simulink model "TestModel2"  (R2012b)
settings: Solver=ode45  SolverMode=SingleTasking  StartTime=0.0  StopTime=10.0  RelTol=1e-3
libraries: simulink x3
settings Model: Creator=odj  LastModifiedBy=TSR2
settings DataIOCC: SignalLoggingSaveFormat=ModelDataLogs
settings OptimizationCC: BlockReduction=off  BooleanDataType=off
settings DebuggingCC: SaveWithParameterizedLinksMsg=none  SignalResolutionControl=TryResolveAllWithWarning  SolverPrmCheckMsg=none  MultiTaskDSMMsg=warning  MultiTaskCondExecSysMsg=none  StrictBusMsg=None
settings HardwareCC: TargetIntDivRoundTo=Zero  TargetEndianess=LittleEndian  TargetHWDeviceType=MATLAB Host  ProdEqTarget=off
settings RTWCC: SystemTargetFile=rtwsfcnfmi.tlc  TemplateMakefile=rtwsfcnfmi_tmf  Description=S-Function Target with Functional Mockup Interface (FMI)  ProcessScript=rtwsfcnfmi_make_rtw_hook  IncludeERTFirstTime=on
settings STFCustomTargetCC: CodeReplacementLibrary=ANSI_C  ModelReferenceCompliant=off  CompOptLevelCompliant=on  GeneratePreprocessorConditionals=Disable all  SystemTargetFile=rtwsfcnfmi.tlc

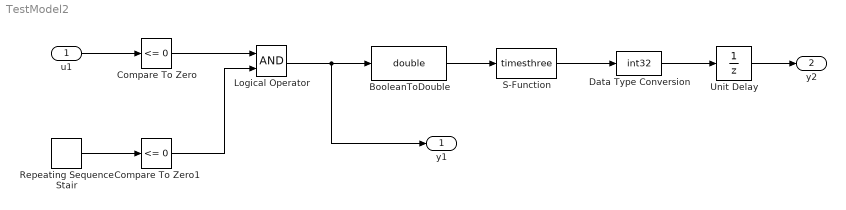
== system TestModel2 ==
  u1 : Inport
  BooleanToDouble : DataTypeConversion  OutDataTypeStr=double
  Compare To Zero : simulink/Logic and Bit Operations/Compare To Zero  relop=<=  OutDataTypeStr=boolean
  Compare To Zero1 : simulink/Logic and Bit Operations/Compare To Zero  relop=<=  OutDataTypeStr=boolean
  Data Type Conversion : DataTypeConversion  OutDataTypeStr=int32
  Logical Operator : Logic  AllPortsSameDT=off  OutDataTypeStr=boolean
  Repeating Sequence Stair : simulink/Sources/Repeating Sequence Stair  OutValues=[3 1 4 2 1].'  tsamp=-1  OutMin=[]  OutMax=[]  OutDataTypeStr=double  OutputDataTypeScalingMode=double  OutDataType=fixdt(0,8)  ConRadixGroup=Best Precision: Vector-wise  OutScaling=2^-12
  S-Function : S-Function  FunctionName=timesthree  EnableBusSupport=off
  Unit Delay : UnitDelay  SampleTime=0.1
  y1 : Outport
  y2 : Outport  Port=2
  wires:
  u1/1 -> Compare To Zero/1
  Compare To Zero1/1 -> Logical Operator/2
  Compare To Zero/1 -> Logical Operator/1
  Unit Delay/1 -> y2/1
  Repeating Sequence Stair/1 -> Compare To Zero1/1
  Logical Operator/1 -> y1/1, BooleanToDouble/1
  BooleanToDouble/1 -> S-Function/1
  S-Function/1 -> Data Type Conversion/1
  Data Type Conversion/1 -> Unit Delay/1
